simulink model "pv_boost_dcac_averaged"  (Simulink 6.5)
settings: Solver=ode45  StartTime=0.0  StopTime=1/60  MaxStep=0.1e-3  RelTol=1e-3
libraries: simulink x6
settings Model: Creator=Mama  LastModifiedBy=Mama
settings DebuggingCC: AlgebraicLoopMsg=none  SolverPrmCheckMsg=none  UnconnectedOutputMsg=none

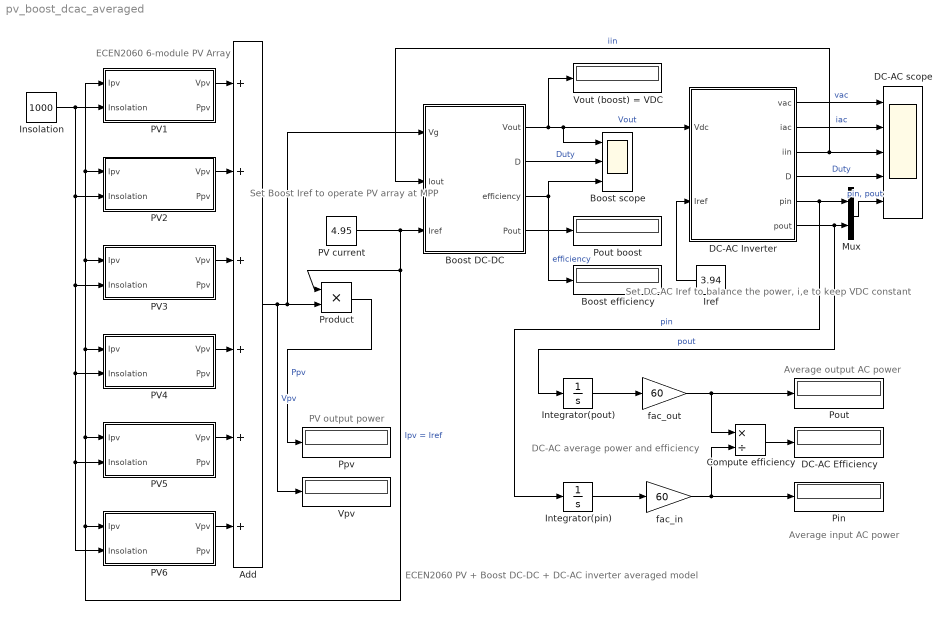
== system pv_boost_dcac_averaged ==
  note: ECEN2060
      | PV + Boost DC-DC + DC-AC inverter averaged model
  note: ECEN2060
      | 6-module PV Array
  note: Average output AC power
  note: Average input AC power
  note: DC-AC average power
      | and efficiency
  note: Set Boost Iref to
      | operate PV array
      | at MPP
  note: Set DC-AC Iref
      | to balance
      | the power, i,e
      | to keep VDC
      | constant
  note: PV output power
  Add : Sum  Inputs=++++++  OutScaling=2^-10
  Boost DC-DC : Subsystem  mask{C=200e-6, Vo=200, RL=0.5, IQ=0.03}
      mask prompts: C "Capacitance"; Vo "Initial capacitor voltage"; RL "Input port series resistance"; IQ "Switching loss current"
      mask help: Averaged model of a boost (step-up) DC-DC converter with input current control. Model includes losses due to input port resistance and output-port switching-loss current.
      mask Display:
      | text(0.5,0.9,'Boost','horizontalAlignment', 'center');
      | text(0.5,0.8,'DC-DC','horizontalAlignment', 'center');
      | text(0.5,0.7,'(averaged, C)','horizontalAlignment', 'center');
      | text(0.5,0.6,'current control','horizontalAlignment', 'center');
  Boost efficiency : Display
  Boost scope : Scope  NumInputPorts=3
      settings: TimeRange=0.018  YMin=180~0.4~0.963  YMax=220~0.6000000000000001~0.967
  Compute efficiency : Product  Inputs=*/  OutScaling=2^-10
  DC-AC scope : Scope  NumInputPorts=5
      settings: TimeRange=0.018  YMin=-200~-10~0~0~0  YMax=200~10~5~1~1000
  DC-AC Efficiency : Display
  DC-AC Inverter : Subsystem  mask{Vrms=120, f=60, RL=0.8, IQ=0.04}
      mask prompts: Vrms "AC line RMS voltage"; f "AC line frequency"; RL "Output port series resistance"; IQ "Switching loss current"
      mask help: Averaged model of a switched-mode DC-AC inverter for single-phase grid-connected systems. Output current is in phase with the AC line voltage and has the RMS value set by the input reference Iref. Conduction losses are modeled by an output por series resistance. Switching losses are modeled by an input port current Isw.
      mask Display:
      | text(0.5,0.75,'DC-AC','horizontalAlignment', 'center');
      | text(0.5,0.6,'inverter','horizontalAlignment', 'center');
      | text(0.5,0.45,'(averaged)','horizontalAlignment', 'center');
  Insolation : Constant  Value=1000  OutDataType=sfix(16)  ConRadixGroup=Use specified scaling  OutScaling=2^0  SampleTime=inf  FramePeriod=inf
  Integrator(pin) : Integrator
  Integrator(pout) : Integrator
  Iref : Constant  Orientation=left  Value=3.94  OutDataType=sfix(16)  ConRadixGroup=Use specified scaling  OutScaling=2^0  SampleTime=inf  FramePeriod=inf
  Mux : Mux  Inputs=2
  PV current : Constant  Value=4.95  OutDataType=sfix(16)  ConRadixGroup=Use specified scaling  OutScaling=2^0  SampleTime=inf  FramePeriod=inf
  PV1 : Subsystem  mask{Isc=5.45, Voc=22.2, Ir=4.95, Vr=17.2, Diode=on}
      mask prompts: Isc "Short-circuit current"; Voc "Open-circuit voltage"; Ir "Current at Pmax"; Vr "Voltage at Pmax"; Diode "By-pass diode?"
      mask help: PV module model based on module data-sheet parameters. This model has Ipv input, which is suitable for series connections. Limitations: no temperature dependance, static model
      mask init:
      | % calculation of PV module parameters
      | % limitation: constant temperature
      | Ns = round(Voc/0.61); % default number of cells in series
      | Vt = 26e-3; % thermal voltage
      | G = Isc/1000; % irradiation to short-circuit current gain
      | Vmpc = Vr/Ns; % cell voltage at rated Pmax
      | Vocc = Voc/Ns; % cell open-circuit voltage
      | Rmpp = Vmpc/Ir; % cell load resistance at Pmax
      | %
      | Rp = 100*Vocc/Isc; % initial value for Rp
      | Vdm = Vocc; % initial value for Vdm
      | %
      | % iterative solution for model parameters: Io, Rs, Rp
      | for i=1:10
      | %
      |  Idm = Isc - Ir - Vdm/Rp; % pn-junction (diode) current at MPP
      |  Io = (Isc-Vocc/Rp)/(exp(Vocc/Vt)-1); % pn-junction reverse saturation current
      |  Vdm = Vt*log(Idm/Io+1); % pn-junction (diode) voltage at MPP
      |  Rs = (Vdm-Vmpc)/Ir; % cell series resistance
      |  Rd = (Rmpp - Rs)*Rp/(Rp-Rmpp+Rs); % diode incremental resistance at MPP
      |  Idm = Vt/Rd; % diode current at MPP based on incremental resistance
      |  Rp = Vdm/(Isc-Ir-Idm); % cell parallel resistance
      | %
      | end
      | %
      mask Display:
      | plot([0.3 0.4],[0.4 0.8]);
      | plot([0.4 0.5],[0.4 0.8]);
      | plot([0.5 0.6],[0.4 0.8]);
      | plot([0.6 0.7],[0.4 0.8]);
      | plot([0.3 0.6],[0.4 0.4]);
      | plot([0.325 0.625],[0.5 0.5]);
      | plot([0.35 0.65],[0.6 0.6]);
      | plot([0.375 0.675],[0.7 0.7]);
      | plot([0.4 0.7],[0.8 0.8]);
      | text(0.5,0.9,'PV module (I)','horizontalAlignment', 'center');
  PV2 : Subsystem  mask{Isc=5.45, Voc=22.2, Ir=4.95, Vr=17.2, Diode=on}
      mask prompts: Isc "Short-circuit current"; Voc "Open-circuit voltage"; Ir "Current at Pmax"; Vr "Voltage at Pmax"; Diode "By-pass diode?"
      mask help: PV module model based on module data-sheet parameters. This model has Ipv input, which is suitable for series connections. Limitations: no temperature dependance, static model
      mask init: same as pv_boost_dcac_averaged/PV1
      mask Display:
      | plot([0.3 0.4],[0.4 0.8]);
      | plot([0.4 0.5],[0.4 0.8]);
      | plot([0.5 0.6],[0.4 0.8]);
      | plot([0.6 0.7],[0.4 0.8]);
      | plot([0.3 0.6],[0.4 0.4]);
      | plot([0.325 0.625],[0.5 0.5]);
      | plot([0.35 0.65],[0.6 0.6]);
      | plot([0.375 0.675],[0.7 0.7]);
      | plot([0.4 0.7],[0.8 0.8]);
      | text(0.5,0.9,'PV module (I)','horizontalAlignment', 'center');
  PV3 : Subsystem  mask{Isc=5.45, Voc=22.2, Ir=4.95, Vr=17.2, Diode=on}
      mask prompts: Isc "Short-circuit current"; Voc "Open-circuit voltage"; Ir "Current at Pmax"; Vr "Voltage at Pmax"; Diode "By-pass diode?"
      mask help: PV module model based on module data-sheet parameters. This model has Ipv input, which is suitable for series connections. Limitations: no temperature dependance, static model
      mask init: same as pv_boost_dcac_averaged/PV1
      mask Display:
      | plot([0.3 0.4],[0.4 0.8]);
      | plot([0.4 0.5],[0.4 0.8]);
      | plot([0.5 0.6],[0.4 0.8]);
      | plot([0.6 0.7],[0.4 0.8]);
      | plot([0.3 0.6],[0.4 0.4]);
      | plot([0.325 0.625],[0.5 0.5]);
      | plot([0.35 0.65],[0.6 0.6]);
      | plot([0.375 0.675],[0.7 0.7]);
      | plot([0.4 0.7],[0.8 0.8]);
      | text(0.5,0.9,'PV module (I)','horizontalAlignment', 'center');
  PV4 : Subsystem  mask{Isc=5.45, Voc=22.2, Ir=4.95, Vr=17.2, Diode=on}
      mask prompts: Isc "Short-circuit current"; Voc "Open-circuit voltage"; Ir "Current at Pmax"; Vr "Voltage at Pmax"; Diode "By-pass diode?"
      mask help: PV module model based on module data-sheet parameters. This model has Ipv input, which is suitable for series connections. Limitations: no temperature dependance, static model
      mask init: same as pv_boost_dcac_averaged/PV1
      mask Display:
      | plot([0.3 0.4],[0.4 0.8]);
      | plot([0.4 0.5],[0.4 0.8]);
      | plot([0.5 0.6],[0.4 0.8]);
      | plot([0.6 0.7],[0.4 0.8]);
      | plot([0.3 0.6],[0.4 0.4]);
      | plot([0.325 0.625],[0.5 0.5]);
      | plot([0.35 0.65],[0.6 0.6]);
      | plot([0.375 0.675],[0.7 0.7]);
      | plot([0.4 0.7],[0.8 0.8]);
      | text(0.5,0.9,'PV module (I)','horizontalAlignment', 'center');
  PV5 : Subsystem  mask{Isc=5.45, Voc=22.2, Ir=4.95, Vr=17.2, Diode=on}
      mask prompts: Isc "Short-circuit current"; Voc "Open-circuit voltage"; Ir "Current at Pmax"; Vr "Voltage at Pmax"; Diode "By-pass diode?"
      mask help: PV module model based on module data-sheet parameters. This model has Ipv input, which is suitable for series connections. Limitations: no temperature dependance, static model
      mask init: same as pv_boost_dcac_averaged/PV1
      mask Display:
      | plot([0.3 0.4],[0.4 0.8]);
      | plot([0.4 0.5],[0.4 0.8]);
      | plot([0.5 0.6],[0.4 0.8]);
      | plot([0.6 0.7],[0.4 0.8]);
      | plot([0.3 0.6],[0.4 0.4]);
      | plot([0.325 0.625],[0.5 0.5]);
      | plot([0.35 0.65],[0.6 0.6]);
      | plot([0.375 0.675],[0.7 0.7]);
      | plot([0.4 0.7],[0.8 0.8]);
      | text(0.5,0.9,'PV module (I)','horizontalAlignment', 'center');
  PV6 : Subsystem  mask{Isc=5.45, Voc=22.2, Ir=4.95, Vr=17.2, Diode=on}
      mask prompts: Isc "Short-circuit current"; Voc "Open-circuit voltage"; Ir "Current at Pmax"; Vr "Voltage at Pmax"; Diode "By-pass diode?"
      mask help: PV module model based on module data-sheet parameters. This model has Ipv input, which is suitable for series connections. Limitations: no temperature dependance, static model
      mask init: same as pv_boost_dcac_averaged/PV1
      mask Display:
      | plot([0.3 0.4],[0.4 0.8]);
      | plot([0.4 0.5],[0.4 0.8]);
      | plot([0.5 0.6],[0.4 0.8]);
      | plot([0.6 0.7],[0.4 0.8]);
      | plot([0.3 0.6],[0.4 0.4]);
      | plot([0.325 0.625],[0.5 0.5]);
      | plot([0.35 0.65],[0.6 0.6]);
      | plot([0.375 0.675],[0.7 0.7]);
      | plot([0.4 0.7],[0.8 0.8]);
      | text(0.5,0.9,'PV module (I)','horizontalAlignment', 'center');
  Pin : Display
  Pout : Display
  Pout boost : Display
  Ppv : Display
  Product : Product  RndMeth=Zero
  Vout (boost) = VDC : Display
  Vpv : Display
  fac_in : Gain  Gain=60
  fac_out : Gain  Gain=60
  wires:
  DC-AC Inverter/1(vac) -> DC-AC scope/1  "vac"
  DC-AC Inverter/2(iac) -> DC-AC scope/2  "iac"
  DC-AC Inverter/3(iin) -> DC-AC scope/3, Boost DC-DC/2(Iout)  "iin"
  DC-AC Inverter/4(D) -> DC-AC scope/4  "Duty"
  DC-AC Inverter/5(pin) -> Integrator(pin)/1, Mux/1  "pin"
  DC-AC Inverter/6(pout) -> Integrator(pout)/1, Mux/2  "pout"
  Integrator(pout)/1 -> fac_out/1
  Integrator(pin)/1 -> fac_in/1
  Compute efficiency/1 -> DC-AC Efficiency/1
  fac_out/1 -> Pout/1, Compute efficiency/1
  fac_in/1 -> Pin/1, Compute efficiency/2
  Boost DC-DC/1(Vout) -> DC-AC Inverter/1(Vdc), Boost scope/1, Vout (boost) = VDC/1  "Vout"
  PV1/1(Vpv) -> Add/1
  PV2/1(Vpv) -> Add/2
  PV3/1(Vpv) -> Add/3
  PV4/1(Vpv) -> Add/4
  PV5/1(Vpv) -> Add/5
  PV6/1(Vpv) -> Add/6
  Add/1 -> Vpv/1, Boost DC-DC/1(Vg), Product/2  "Vpv"
  Insolation/1 -> PV5/2(Insolation), PV6/2(Insolation), PV4/2(Insolation), PV3/2(Insolation), PV2/2(Insolation), PV1/2(Insolation)
  Iref/1 -> DC-AC Inverter/2(Iref)
  Product/1 -> Ppv/1  "Ppv"
  PV current/1 -> Boost DC-DC/3(Iref), PV1/1(Ipv), PV2/1(Ipv), PV3/1(Ipv), PV4/1(Ipv), PV5/1(Ipv), PV6/1(Ipv), Product/1  "Ipv = Iref"
  Boost DC-DC/2(D) -> Boost scope/2  "Duty"
  Boost DC-DC/3(efficiency) -> Boost scope/3, Boost efficiency/1  "efficiency"
  Boost DC-DC/4(Pout) -> Pout boost/1
  Mux/1 -> DC-AC scope/5  "pin, pout"

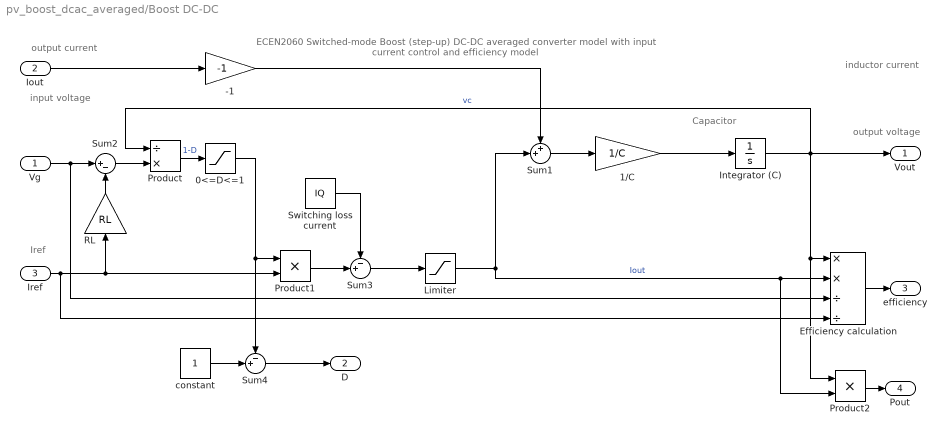
== system pv_boost_dcac_averaged/Boost DC-DC ==
  note: ECEN2060 Switched-mode Boost (step-up) DC-DC averaged converter model
      | with input current control and efficiency model
  note: output voltage
  note: inductor current
  note: output current
  note: input voltage
  note: Iref
  note: Capacitor
  Vg : Inport
  Iout : Inport  Port=2
  Iref : Inport  Port=3
  -1 : Gain  Gain=-1
  0<=D<=1 : Saturate  UpperLimit=1  LowerLimit=0
  1/C : Gain  Gain=1/C
  Efficiency calculation : Product  Inputs=**//  RndMeth=Zero
  Integrator (C) : Integrator  InitialCondition=Vo
  Limiter : Saturate  UpperLimit=inf  LowerLimit=0
  Product : Product  Inputs=/*  RndMeth=Zero
  Product1 : Product  Inputs=**  RndMeth=Zero
  Product2 : Product  Inputs=**  RndMeth=Zero
  RL : Gain  Orientation=up  Gain=RL
  Sum1 : Sum  Inputs=++|
  Sum2 : Sum  Inputs=|+-
  Sum3 : Sum  Inputs=-+|
  Sum4 : Sum  Inputs=-+|
  Switching loss current : Constant  Value=IQ  OutDataType=sfix(16)  ConRadixGroup=Use specified scaling  OutScaling=2^0  SampleTime=inf  FramePeriod=inf
  constant : Constant  Value=1  OutDataType=sfix(16)  ConRadixGroup=Use specified scaling  OutScaling=2^0  SampleTime=inf  FramePeriod=inf
  Vout : Outport
  D : Outport  Port=2
  efficiency : Outport  Port=3
  Pout : Outport  Port=4
  wires:
  Sum1/1 -> 1/C/1
  1/C/1 -> Integrator (C)/1
  Integrator (C)/1 -> Vout/1, Product/1, Efficiency calculation/1, Product2/1  "vc"
  Iout/1 -> -1/1
  -1/1 -> Sum1/1
  RL/1 -> Sum2/2
  Iref/1 -> RL/1, Product1/2, Efficiency calculation/4
  Vg/1 -> Sum2/1, Efficiency calculation/3
  Sum2/1 -> Product/2
  Product1/1 -> Sum3/2
  Switching loss current/1 -> Sum3/1
  Sum3/1 -> Limiter/1
  Limiter/1 -> Sum1/2, Efficiency calculation/2, Product2/2  "Iout"
  Efficiency calculation/1 -> efficiency/1
  constant/1 -> Sum4/2
  Sum4/1 -> D/1
  Product2/1 -> Pout/1
  Product/1 -> 0<=D<=1/1  "1-D"
  0<=D<=1/1 -> Product1/1, Sum4/1

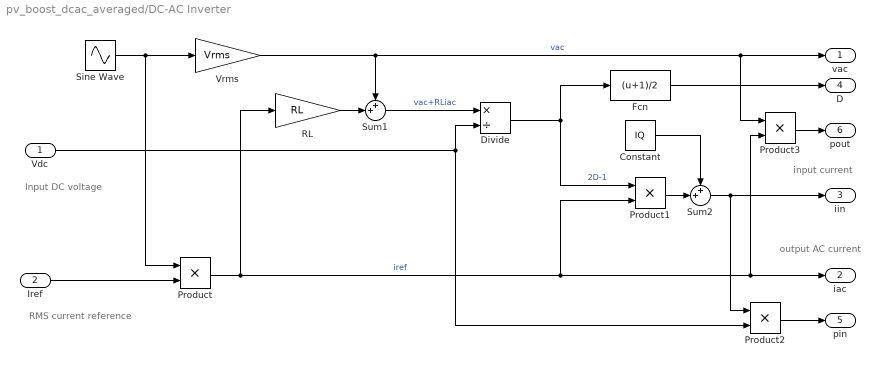
== system pv_boost_dcac_averaged/DC-AC Inverter ==
  note: output AC current
  note: Input DC voltage
  note: RMS current reference
  note: input current
  Vdc : Inport
  Iref : Inport  Port=2
  Constant : Constant  Value=IQ  OutDataType=sfix(16)  ConRadixGroup=Use specified scaling  OutScaling=2^0  SampleTime=inf  FramePeriod=inf
  Divide : Product  Inputs=*/  OutScaling=2^-10
  Fcn : Fcn  Expr=(u+1)/2
  Product{,1..3} (4 alike) : Product  RndMeth=Zero
  RL : Gain  Gain=RL
  Sine Wave : Sin  Amplitude=1*sqrt(2)  Frequency=2*pi*f  SampleTime=0
  Sum1 : Sum  Inputs=++|
  Sum2 : Sum  Inputs=++|
  Vrms : Gain  Gain=Vrms
  vac : Outport
  iac : Outport  Port=2
  iin : Outport  Port=3
  D : Outport  Port=4
  pin : Outport  Port=5
  pout : Outport  Port=6
  wires:
  Sine Wave/1 -> Vrms/1, Product/1
  Vrms/1 -> Sum1/1, vac/1, Product3/1  "vac"
  Product/1 -> RL/1, Product1/2, iac/1, Product3/2  "iref"
  Iref/1 -> Product/2
  RL/1 -> Sum1/2
  Sum1/1 -> Divide/1  "vac+RLiac"
  Vdc/1 -> Divide/2, Product2/2
  Divide/1 -> Product1/1, Fcn/1  "2D-1"
  Product1/1 -> Sum2/2
  Constant/1 -> Sum2/1
  Sum2/1 -> Product2/1, iin/1
  Fcn/1 -> D/1
  Product2/1 -> pin/1
  Product3/1 -> pout/1

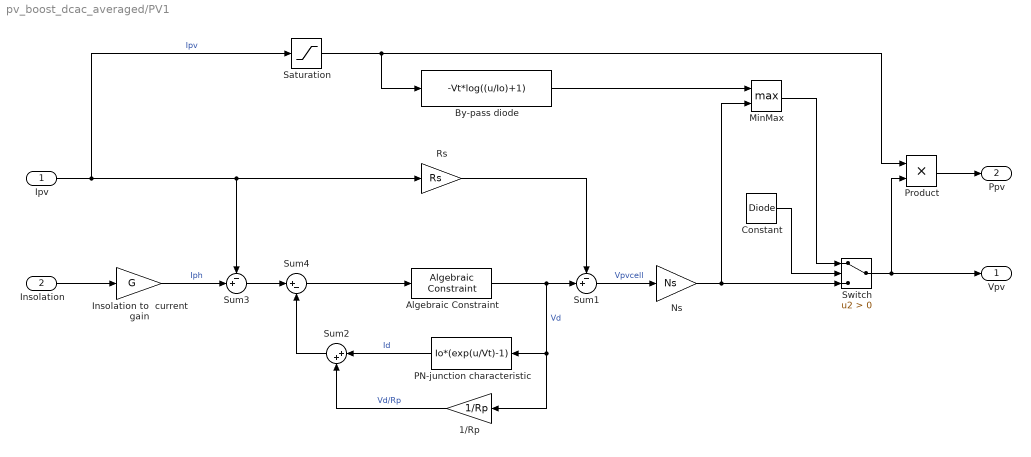
== system pv_boost_dcac_averaged/PV1 ==
  Ipv : Inport
  Insolation : Inport  Port=2
  1/Rp : Gain  Orientation=left  Gain=1/Rp
  Algebraic Constraint : simulink/Math Operations/Algebraic Constraint  SystemSampleTime=-1  z0=0
  By-pass diode : Fcn  Expr=-Vt*log((u/Io)+1)
  Constant : Constant  Value=Diode  OutDataType=sfix(16)  ConRadixGroup=Use specified scaling  OutScaling=2^0  SampleTime=inf  FramePeriod=inf
  Insolation to  current gain : Gain  Gain=G
  MinMax : MinMax  Function=max  Inputs=2
  Ns : Gain  Gain=Ns
  PN-junction characteristic : Fcn  Orientation=left  Expr=Io*(exp(u/Vt)-1)
  Product : Product  RndMeth=Zero
  Rs : Gain  Gain=Rs
  Saturation : Saturate  UpperLimit=inf  LowerLimit=0
  Sum1 : Sum  Inputs=-+|
  Sum2 : Sum  Orientation=left  Inputs=|++
  Sum3 : Sum  Inputs=-+|
  Sum4 : Sum  Inputs=|+-
  Switch : Switch  Criteria=u2 > Threshold
  Vpv : Outport
  Ppv : Outport  Port=2
  wires:
  Insolation/1 -> Insolation to  current gain/1
  Insolation to  current gain/1 -> Sum3/2  "Iph"
  Ipv/1 -> Saturation/1, Sum3/1, Rs/1  "Ipv"
  Product/1 -> Ppv/1
  Sum4/1 -> Algebraic Constraint/1
  Algebraic Constraint/1 -> Sum1/2, 1/Rp/1, PN-junction characteristic/1  "Vd"
  Sum1/1 -> Ns/1  "Vpvcell"
  Rs/1 -> Sum1/1
  By-pass diode/1 -> MinMax/1
  Ns/1 -> MinMax/2, Switch/3
  MinMax/1 -> Switch/1
  Constant/1 -> Switch/2
  Switch/1 -> Vpv/1, Product/2
  Saturation/1 -> Product/1, By-pass diode/1
  Sum3/1 -> Sum4/1
  Sum2/1 -> Sum4/2
  PN-junction characteristic/1 -> Sum2/1  "Id"
  1/Rp/1 -> Sum2/2  "Vd/Rp"

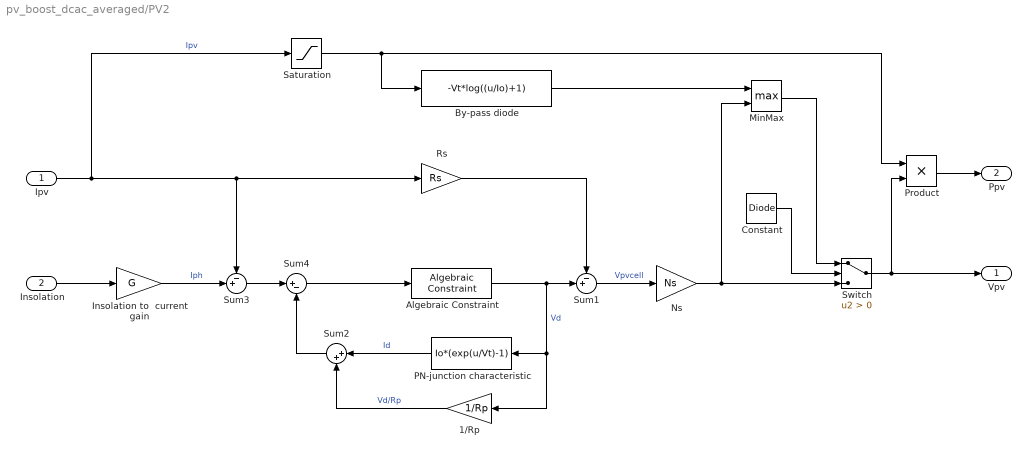
== system pv_boost_dcac_averaged/PV2 ==
  Ipv : Inport
  Insolation : Inport  Port=2
  1/Rp : Gain  Orientation=left  Gain=1/Rp
  Algebraic Constraint : simulink/Math Operations/Algebraic Constraint  SystemSampleTime=-1  z0=0
  By-pass diode : Fcn  Expr=-Vt*log((u/Io)+1)
  Constant : Constant  Value=Diode  OutDataType=sfix(16)  ConRadixGroup=Use specified scaling  OutScaling=2^0  SampleTime=inf  FramePeriod=inf
  Insolation to  current gain : Gain  Gain=G
  MinMax : MinMax  Function=max  Inputs=2
  Ns : Gain  Gain=Ns
  PN-junction characteristic : Fcn  Orientation=left  Expr=Io*(exp(u/Vt)-1)
  Product : Product  RndMeth=Zero
  Rs : Gain  Gain=Rs
  Saturation : Saturate  UpperLimit=inf  LowerLimit=0
  Sum1 : Sum  Inputs=-+|
  Sum2 : Sum  Orientation=left  Inputs=|++
  Sum3 : Sum  Inputs=-+|
  Sum4 : Sum  Inputs=|+-
  Switch : Switch  Criteria=u2 > Threshold
  Vpv : Outport
  Ppv : Outport  Port=2
  wires:
  Insolation/1 -> Insolation to  current gain/1
  Insolation to  current gain/1 -> Sum3/2  "Iph"
  Ipv/1 -> Saturation/1, Sum3/1, Rs/1  "Ipv"
  Product/1 -> Ppv/1
  Sum4/1 -> Algebraic Constraint/1
  Algebraic Constraint/1 -> Sum1/2, 1/Rp/1, PN-junction characteristic/1  "Vd"
  Sum1/1 -> Ns/1  "Vpvcell"
  Rs/1 -> Sum1/1
  By-pass diode/1 -> MinMax/1
  Ns/1 -> MinMax/2, Switch/3
  MinMax/1 -> Switch/1
  Constant/1 -> Switch/2
  Switch/1 -> Vpv/1, Product/2
  Saturation/1 -> Product/1, By-pass diode/1
  Sum3/1 -> Sum4/1
  Sum2/1 -> Sum4/2
  PN-junction characteristic/1 -> Sum2/1  "Id"
  1/Rp/1 -> Sum2/2  "Vd/Rp"

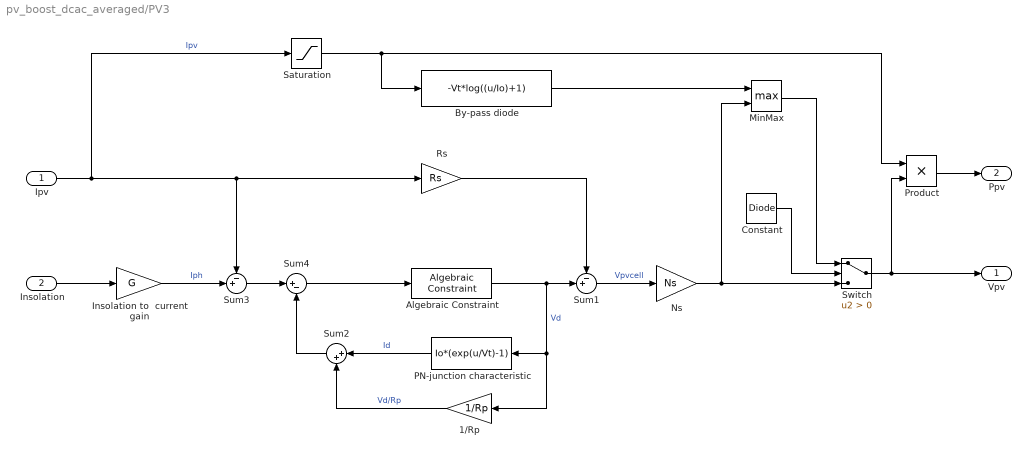
== system pv_boost_dcac_averaged/PV3 ==
  Ipv : Inport
  Insolation : Inport  Port=2
  1/Rp : Gain  Orientation=left  Gain=1/Rp
  Algebraic Constraint : simulink/Math Operations/Algebraic Constraint  SystemSampleTime=-1  z0=0
  By-pass diode : Fcn  Expr=-Vt*log((u/Io)+1)
  Constant : Constant  Value=Diode  OutDataType=sfix(16)  ConRadixGroup=Use specified scaling  OutScaling=2^0  SampleTime=inf  FramePeriod=inf
  Insolation to  current gain : Gain  Gain=G
  MinMax : MinMax  Function=max  Inputs=2
  Ns : Gain  Gain=Ns
  PN-junction characteristic : Fcn  Orientation=left  Expr=Io*(exp(u/Vt)-1)
  Product : Product  RndMeth=Zero
  Rs : Gain  Gain=Rs
  Saturation : Saturate  UpperLimit=inf  LowerLimit=0
  Sum1 : Sum  Inputs=-+|
  Sum2 : Sum  Orientation=left  Inputs=|++
  Sum3 : Sum  Inputs=-+|
  Sum4 : Sum  Inputs=|+-
  Switch : Switch  Criteria=u2 > Threshold
  Vpv : Outport
  Ppv : Outport  Port=2
  wires:
  Insolation/1 -> Insolation to  current gain/1
  Insolation to  current gain/1 -> Sum3/2  "Iph"
  Ipv/1 -> Saturation/1, Sum3/1, Rs/1  "Ipv"
  Product/1 -> Ppv/1
  Sum4/1 -> Algebraic Constraint/1
  Algebraic Constraint/1 -> Sum1/2, 1/Rp/1, PN-junction characteristic/1  "Vd"
  Sum1/1 -> Ns/1  "Vpvcell"
  Rs/1 -> Sum1/1
  By-pass diode/1 -> MinMax/1
  Ns/1 -> MinMax/2, Switch/3
  MinMax/1 -> Switch/1
  Constant/1 -> Switch/2
  Switch/1 -> Vpv/1, Product/2
  Saturation/1 -> Product/1, By-pass diode/1
  Sum3/1 -> Sum4/1
  Sum2/1 -> Sum4/2
  PN-junction characteristic/1 -> Sum2/1  "Id"
  1/Rp/1 -> Sum2/2  "Vd/Rp"

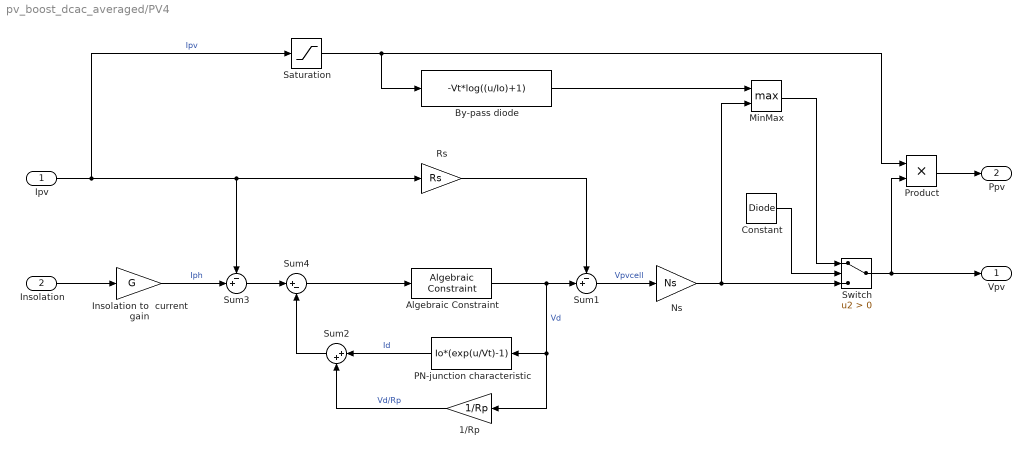
== system pv_boost_dcac_averaged/PV4 ==
  Ipv : Inport
  Insolation : Inport  Port=2
  1/Rp : Gain  Orientation=left  Gain=1/Rp
  Algebraic Constraint : simulink/Math Operations/Algebraic Constraint  SystemSampleTime=-1  z0=0
  By-pass diode : Fcn  Expr=-Vt*log((u/Io)+1)
  Constant : Constant  Value=Diode  OutDataType=sfix(16)  ConRadixGroup=Use specified scaling  OutScaling=2^0  SampleTime=inf  FramePeriod=inf
  Insolation to  current gain : Gain  Gain=G
  MinMax : MinMax  Function=max  Inputs=2
  Ns : Gain  Gain=Ns
  PN-junction characteristic : Fcn  Orientation=left  Expr=Io*(exp(u/Vt)-1)
  Product : Product  RndMeth=Zero
  Rs : Gain  Gain=Rs
  Saturation : Saturate  UpperLimit=inf  LowerLimit=0
  Sum1 : Sum  Inputs=-+|
  Sum2 : Sum  Orientation=left  Inputs=|++
  Sum3 : Sum  Inputs=-+|
  Sum4 : Sum  Inputs=|+-
  Switch : Switch  Criteria=u2 > Threshold
  Vpv : Outport
  Ppv : Outport  Port=2
  wires:
  Insolation/1 -> Insolation to  current gain/1
  Insolation to  current gain/1 -> Sum3/2  "Iph"
  Ipv/1 -> Saturation/1, Sum3/1, Rs/1  "Ipv"
  Product/1 -> Ppv/1
  Sum4/1 -> Algebraic Constraint/1
  Algebraic Constraint/1 -> Sum1/2, 1/Rp/1, PN-junction characteristic/1  "Vd"
  Sum1/1 -> Ns/1  "Vpvcell"
  Rs/1 -> Sum1/1
  By-pass diode/1 -> MinMax/1
  Ns/1 -> MinMax/2, Switch/3
  MinMax/1 -> Switch/1
  Constant/1 -> Switch/2
  Switch/1 -> Vpv/1, Product/2
  Saturation/1 -> Product/1, By-pass diode/1
  Sum3/1 -> Sum4/1
  Sum2/1 -> Sum4/2
  PN-junction characteristic/1 -> Sum2/1  "Id"
  1/Rp/1 -> Sum2/2  "Vd/Rp"

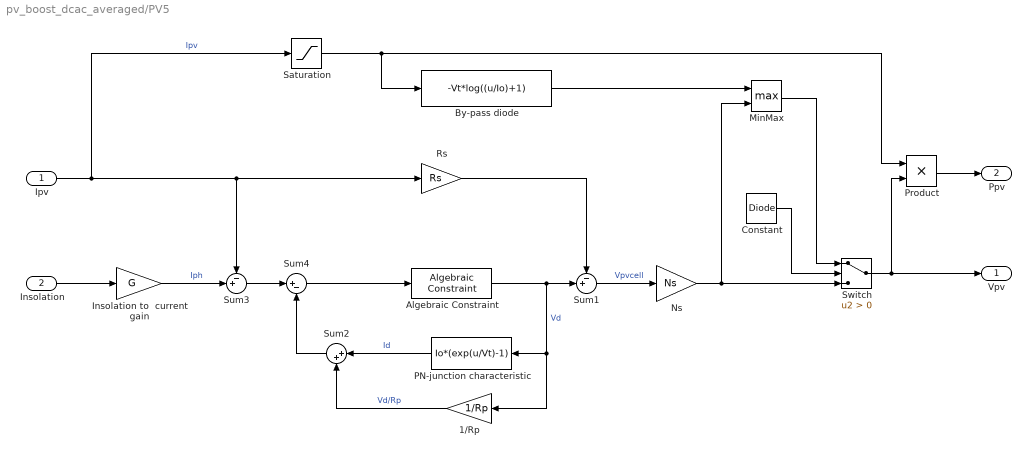
== system pv_boost_dcac_averaged/PV5 ==
  Ipv : Inport
  Insolation : Inport  Port=2
  1/Rp : Gain  Orientation=left  Gain=1/Rp
  Algebraic Constraint : simulink/Math Operations/Algebraic Constraint  SystemSampleTime=-1  z0=0
  By-pass diode : Fcn  Expr=-Vt*log((u/Io)+1)
  Constant : Constant  Value=Diode  OutDataType=sfix(16)  ConRadixGroup=Use specified scaling  OutScaling=2^0  SampleTime=inf  FramePeriod=inf
  Insolation to  current gain : Gain  Gain=G
  MinMax : MinMax  Function=max  Inputs=2
  Ns : Gain  Gain=Ns
  PN-junction characteristic : Fcn  Orientation=left  Expr=Io*(exp(u/Vt)-1)
  Product : Product  RndMeth=Zero
  Rs : Gain  Gain=Rs
  Saturation : Saturate  UpperLimit=inf  LowerLimit=0
  Sum1 : Sum  Inputs=-+|
  Sum2 : Sum  Orientation=left  Inputs=|++
  Sum3 : Sum  Inputs=-+|
  Sum4 : Sum  Inputs=|+-
  Switch : Switch  Criteria=u2 > Threshold
  Vpv : Outport
  Ppv : Outport  Port=2
  wires:
  Insolation/1 -> Insolation to  current gain/1
  Insolation to  current gain/1 -> Sum3/2  "Iph"
  Ipv/1 -> Saturation/1, Sum3/1, Rs/1  "Ipv"
  Product/1 -> Ppv/1
  Sum4/1 -> Algebraic Constraint/1
  Algebraic Constraint/1 -> Sum1/2, 1/Rp/1, PN-junction characteristic/1  "Vd"
  Sum1/1 -> Ns/1  "Vpvcell"
  Rs/1 -> Sum1/1
  By-pass diode/1 -> MinMax/1
  Ns/1 -> MinMax/2, Switch/3
  MinMax/1 -> Switch/1
  Constant/1 -> Switch/2
  Switch/1 -> Vpv/1, Product/2
  Saturation/1 -> Product/1, By-pass diode/1
  Sum3/1 -> Sum4/1
  Sum2/1 -> Sum4/2
  PN-junction characteristic/1 -> Sum2/1  "Id"
  1/Rp/1 -> Sum2/2  "Vd/Rp"

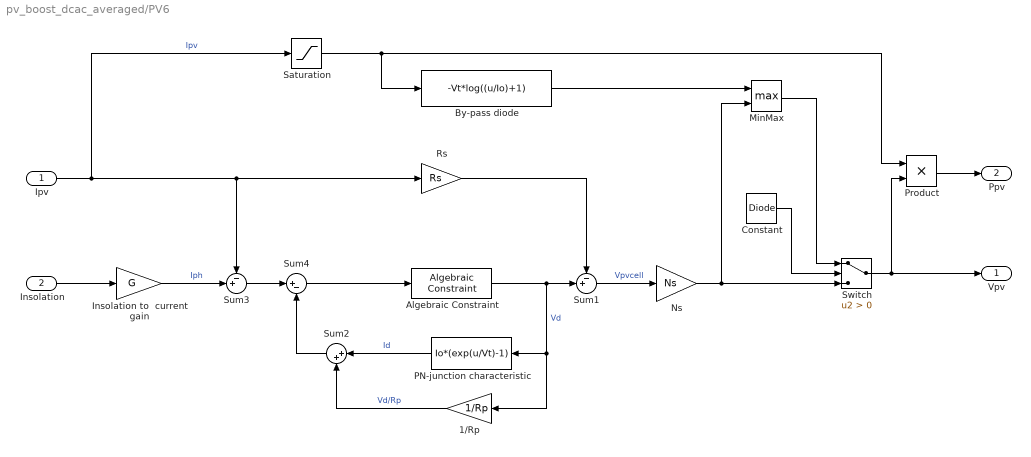
== system pv_boost_dcac_averaged/PV6 ==
  Ipv : Inport
  Insolation : Inport  Port=2
  1/Rp : Gain  Orientation=left  Gain=1/Rp
  Algebraic Constraint : simulink/Math Operations/Algebraic Constraint  SystemSampleTime=-1  z0=0
  By-pass diode : Fcn  Expr=-Vt*log((u/Io)+1)
  Constant : Constant  Value=Diode  OutDataType=sfix(16)  ConRadixGroup=Use specified scaling  OutScaling=2^0  SampleTime=inf  FramePeriod=inf
  Insolation to  current gain : Gain  Gain=G
  MinMax : MinMax  Function=max  Inputs=2
  Ns : Gain  Gain=Ns
  PN-junction characteristic : Fcn  Orientation=left  Expr=Io*(exp(u/Vt)-1)
  Product : Product  RndMeth=Zero
  Rs : Gain  Gain=Rs
  Saturation : Saturate  UpperLimit=inf  LowerLimit=0
  Sum1 : Sum  Inputs=-+|
  Sum2 : Sum  Orientation=left  Inputs=|++
  Sum3 : Sum  Inputs=-+|
  Sum4 : Sum  Inputs=|+-
  Switch : Switch  Criteria=u2 > Threshold
  Vpv : Outport
  Ppv : Outport  Port=2
  wires:
  Insolation/1 -> Insolation to  current gain/1
  Insolation to  current gain/1 -> Sum3/2  "Iph"
  Ipv/1 -> Saturation/1, Sum3/1, Rs/1  "Ipv"
  Product/1 -> Ppv/1
  Sum4/1 -> Algebraic Constraint/1
  Algebraic Constraint/1 -> Sum1/2, 1/Rp/1, PN-junction characteristic/1  "Vd"
  Sum1/1 -> Ns/1  "Vpvcell"
  Rs/1 -> Sum1/1
  By-pass diode/1 -> MinMax/1
  Ns/1 -> MinMax/2, Switch/3
  MinMax/1 -> Switch/1
  Constant/1 -> Switch/2
  Switch/1 -> Vpv/1, Product/2
  Saturation/1 -> Product/1, By-pass diode/1
  Sum3/1 -> Sum4/1
  Sum2/1 -> Sum4/2
  PN-junction characteristic/1 -> Sum2/1  "Id"
  1/Rp/1 -> Sum2/2  "Vd/Rp"
